simulink model "tubulao"  (R2018b)
settings: Solver=ode45  StartTime=0.0  StopTime=100  MaxStep=1e-2  RelTol=1e-3  EnableMultiTasking=on
undefined symbols (not defined in the file): kc_ex, l, magnitude, R, Ti_ex
settings Model: Creator=Pichau  LastModifiedBy=Aniel
settings DataIOCC: LimitDataPoints=on
settings OptimizationCC: LifeSpan=inf
settings DebuggingCC: AllowSymbolicDim=off  SFUnexpectedBacktrackingDiag=warning  SFNoUnconditionalDefaultTransitionDiag=warning  SFExecutionAtInitializationDiag=none
settings ModelReferenceCC: PropagateSignalLabelsOutOfModel=off
settings SFSimCC: SimUseLocalCustomCode=off
settings RTWCC: RTWUseLocalCustomCode=off
settings CodeAppCC: StateflowObjectComments=on
settings GRTTargetCC: TargetLangStandard=C89/C90 (ANSI)
settings ConfigComp: CovMetricSettings=dw  CovHtmlReporting=on  CovSaveCumulativeToWorkspaceVar=on  CovSaveSingleToWorkspaceVar=on  CovExternalEMLEnable=off

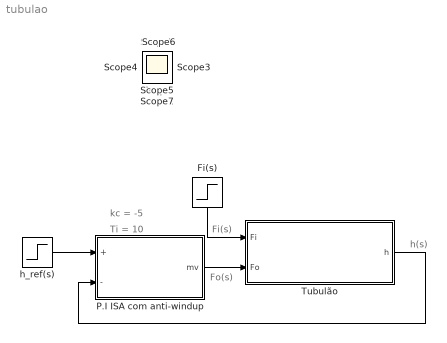
== system tubulao ==
  note: Ti = 10
  note: kc = -5
  note: Fo(s)
  note: Fi(s)
  note: h(s)
  Fi(s) : Step  SampleTime=0
  P.I ISA com anti-windup : Subsystem
  Tubulão : Subsystem
  h_ref(s) : Step  Time=50  Before=R  After=R/2  SampleTime=0
  Scope{,1..7} (8 alike) : Scope
  wires:
  h_ref(s)/1 -> P.I ISA com anti-windup/1(+)
  Fi(s)/1 -> Tubulão/1(Fi)
  Tubulão/1(h) -> P.I ISA com anti-windup/2(-)
  P.I ISA com anti-windup/1(mv) -> Tubulão/2(Fo)

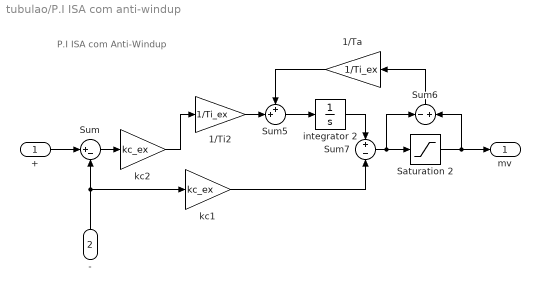
== system tubulao/P.I ISA com anti-windup ==
  note: P.I ISA com Anti-Windup
  + : Inport
  - : Inport  Port=2
  1/Ta : Gain  Gain=1/Ti_ex
  1/Ti2 : Gain  Gain=1/Ti_ex
  Saturation 2 : Saturate  UpperLimit=2  LowerLimit=0
  Sum : Sum  Inputs=|+-
  Sum5 : Sum  Inputs=++|
  Sum6 : Sum  Inputs=-+
  Sum7 : Sum  Inputs=+-
  integrator 2 : Integrator
  kc1 : Gain  Gain=kc_ex
  kc2 : Gain  Gain=kc_ex
  mv : Outport
  wires:
  Sum7/1 -> Sum6/1, Saturation 2/1
  1/Ti2/1 -> Sum5/2
  Sum5/1 -> integrator 2/1
  Saturation 2/1 -> mv/1, Sum6/2
  1/Ta/1 -> Sum5/1
  kc2/1 -> 1/Ti2/1
  Sum6/1 -> 1/Ta/1
  integrator 2/1 -> Sum7/1
  Sum/1 -> kc2/1
  +/1 -> Sum/1
  -/1 -> kc1/1, Sum/2
  kc1/1 -> Sum7/2

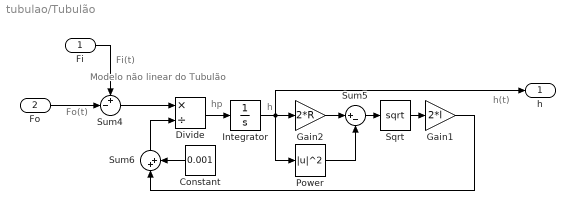
== system tubulao/Tubulão ==
  note: Fo(t)
  note: Modelo não linear do Tubulão
  note: h
  note: h(t)
  note: hp
  note: Fi(t)
  Fi : Inport
  Fo : Inport  Port=2
  Constant : Constant  Value=0.001
  Divide : Product  Inputs=*/
  Gain1 : Gain  Gain=2*l
  Gain2 : Gain  Gain=2*R
  Integrator : Integrator  LimitOutput=on  UpperSaturationLimit=2*R  LowerSaturationLimit=0
  Power : Math  Operator=magnitude^2  SaturateOnIntegerOverflow=on
  Sqrt : Sqrt  SaturateOnIntegerOverflow=on
  Sum4 : Sum  Inputs=+-|
  Sum5 : Sum  Inputs=|+-
  Sum6 : Sum  Inputs=|++
  h : Outport
  wires:
  Fo/1 -> Sum4/2
  Integrator/1 -> Power/1, h/1, Gain2/1
  Constant/1 -> Sum6/2
  Gain2/1 -> Sum5/1
  Gain1/1 -> Sum6/1
  Sqrt/1 -> Gain1/1
  Sum6/1 -> Divide/2
  Sum4/1 -> Divide/1
  Power/1 -> Sum5/2
  Divide/1 -> Integrator/1
  Sum5/1 -> Sqrt/1
  Fi/1 -> Sum4/1
